simulink library "INT_BrkPed_SetData"  (R2016b)
settings: Solver=VariableStepAuto  StartTime=0.0  StopTime=10.0  RelTol=1e-3
settings Model: Creator=Administrator  LastModifiedBy=Administrator

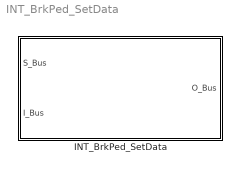
== system INT_BrkPed_SetData ==
  INT_BrkPed_SetData : Subsystem

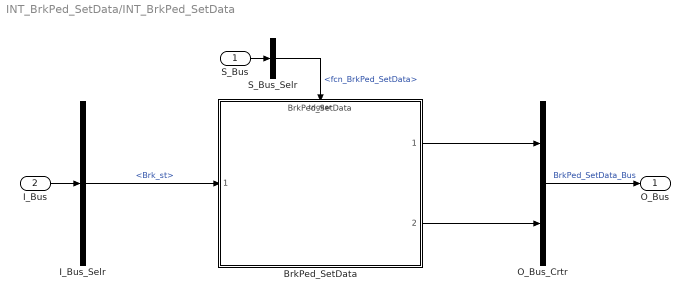
== system INT_BrkPed_SetData/INT_BrkPed_SetData ==
  S_Bus : Inport
  I_Bus : Inport  Port=2
  BrkPed_SetData : ModelReference  ModelNameDialog=BrkPed_SetData  SimulationMode=Normal  ModelReferenceVersion=1.4  TriggerPortName=function  TriggerPortTriggerType=function-call  TriggerPortStatesWhenEnabling=held
  I_Bus_Selr : BusSelector  OutputSignals=Brk_st
  O_Bus_Crtr : BusCreator  Inputs=2
  S_Bus_Selr : BusSelector  OutputSignals=fcn_BrkPed_SetData
  O_Bus : Outport
  wires:
  S_Bus_Selr/1 -> BrkPed_SetData/Trigger  "<fcn_BrkPed_SetData>"
  S_Bus/1 -> S_Bus_Selr/1
  I_Bus/1 -> I_Bus_Selr/1
  I_Bus_Selr/1 -> BrkPed_SetData/1  "<Brk_st>"
  O_Bus_Crtr/1 -> O_Bus/1  "BrkPed_SetData_Bus"
  BrkPed_SetData/1 -> O_Bus_Crtr/1
  BrkPed_SetData/2 -> O_Bus_Crtr/2
